simulink model "test_pwm_main_out_02"  (Simulink 8.8)
settings: Solver=FixedStepDiscrete  StartTime=0.0  StopTime=10.0  FixedStep=0.01  RelTol=1e-3  EnableMultiTasking=on
InitFcn:
  | px4_ap1_mdl_callback('check_model');
libraries: px4_ap1_pwm_main_out_lib x1, px4_ap1_px4setup_lib x1
settings Model: Creator=Privat  LastModifiedBy=Privat
settings OptimizationCC: ExpressionDepthLimit=2147483647  InitFltsAndDblsToZero=on  LifeSpan=1
settings DebuggingCC: SolverPrmCheckMsg=warning  InheritedTsInSrcMsg=none
settings RTWCC: SystemTargetFile=px4_ap1.tlc  GenCodeOnly=on  GenerateMakefile=off
settings CodeAppCC: IgnoreCustomStorageClasses=off  CustomSymbolStrType=$N$R$M  InternalIdentifier=Classic
settings STFCustomTargetCC: ModelReferenceCompliant=off  IncludeMdlTerminateFcn=off  CombineOutputUpdateFcns=on  ERTCustomFileBanners=on  SupportContinuousTime=off  SupportNonInlinedSFcns=off  RemoveResetFunc=on  MATLABClassNameForMDSCustomization=Simulink.SoftwareTarget.ERTCustomization  CPPClassGenCompliant=on  GRTInterface=off  SystemTargetFile=px4_ap1.tlc
settings ERTTargetCC: MultiwordLength=2048  ModelReferenceCompliant=off  ParMdlRefBuildCompliant=off  CompOptLevelCompliant=off  ConcurrentExecutionCompliant=off  IncludeMdlTerminateFcn=off  ERTFirstTimeCompliant=off  ModelStepFunctionPrototypeControlCompliant=off  UseToolchainInfoCompliant=off  ERTSrcFileBannerTemplate=px4_ap1_code_template.cgt  ERTHdrFileBannerTemplate=px4_ap1_code_template.cgt  ERTDataSrcFileTemplate=px4_ap1_code_template.cgt  ERTDataHdrFileTemplate=px4_ap1_code_template.cgt  ERTCustomFileTemplate=px4_ap1_main.tlc  ConvertIfToSwitch=off  SuppressUnreachableDefaultCases=off

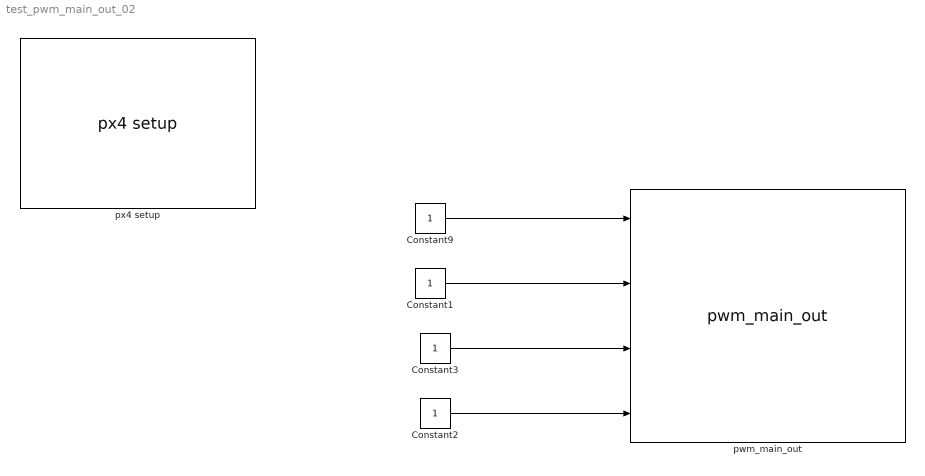
== system test_pwm_main_out_02 ==
  Constant1 : Constant  OutDataTypeStr=boolean
  Constant2 : Constant  OutDataTypeStr=uint16
  Constant3 : Constant  OutDataTypeStr=uint16
  Constant9 : Constant  OutDataTypeStr=boolean
  pwm_main_out : px4_ap1_pwm_main_out_lib/pwm_main_out  Description=Setup for PX4 native software  main1=on  main2=off  main3=off  main4=off  main5=off  main6=off  main7=off  main8=on  def_pwm=50  alt_pwm=400  pwm_1_2=Alternate  pwm_3_4=Alternate  pwm_5_8=Alternate
  px4 setup : px4_ap1_px4setup_lib/px4 setup  SampleTimeValue=0.01  cbBuild=on  cbUpload=off  cbPort=COM0  cpuLoad=on  debugmode=on
  wires:
  Constant9/1 -> pwm_main_out/1
  Constant1/1 -> pwm_main_out/2
  Constant3/1 -> pwm_main_out/3
  Constant2/1 -> pwm_main_out/4
